simulink library "dragTurbine"  (R2022a)
settings: Solver=VariableStepAuto  StartTime=0.0  StopTime=10.0  RelTol=1e-3
undefined symbols (not defined in the file): flwSpd, rho, vcl
libraries: simulink x2, vrlib x2, localApparentWind_ul x1
settings Model: Creator=Ayaz  LastModifiedBy=kavin
settings SolverCC: AlgebraicLoopSolver=TrustRegion
settings DataIOCC: ReturnWorkspaceOutputs=off
settings DebuggingCC: UnconnectedInputMsg=warning  UnconnectedOutputMsg=warning  UnconnectedLineMsg=warning  SFMachineParentedDataDiag=warning  ArithmeticOperatorsInVariantConditions=warning
settings SFSimCC: CustomCodeUndefinedFunction=UseInterfaceOnly

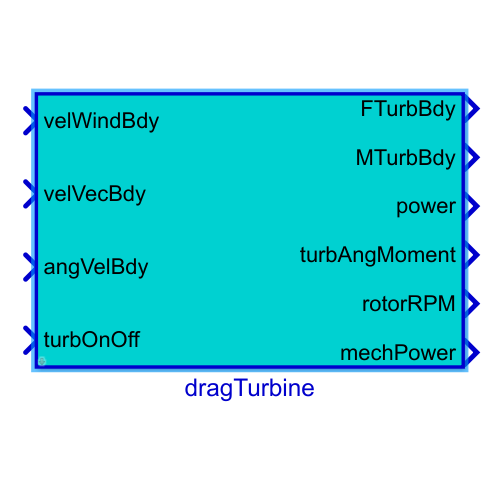
[thumbnail: Simulink's stored preview of the top-level diagram]
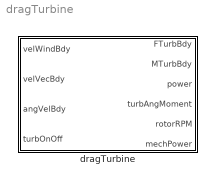
== system dragTurbine ==
  dragTurbine : Subsystem  TreatAsAtomicUnit=on  mask{vhcl=vcl, thr=0}
      mask prompts: vhcl "Vehicle Object"; thr "Tether Object"

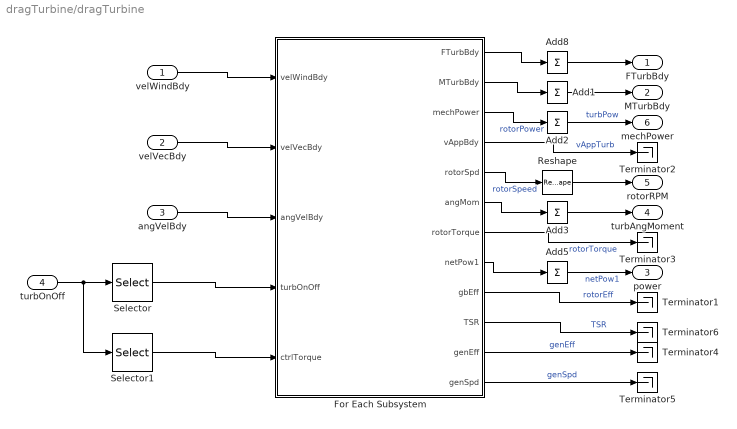
== system dragTurbine/dragTurbine ==
  velWindBdy : Inport
  velVecBdy : Inport  Port=2
  angVelBdy : Inport  Port=3
  turbOnOff : Inport  Port=4
  Add{1..3,8} (4 alike) : Sum  Inputs=1  CollapseMode=Specified dimension  CollapseDim=2
  Add5 : Sum  Inputs=1  CollapseDim=2
  For Each Subsystem : Subsystem  TreatAsAtomicUnit=on  mask{rho=rho, turb_struct=vhcl.struct('OCT.turb'), vhcl=vhcl}
      mask prompts: rho "Fluid Density"; turb_struct "Turbine Structure"; vhcl "Vehicle"
      settings: MinAlgLoopOccurrences=on
  Reshape : Reshape  OutputDimensionality=Column vector (2-D)
  Selector : Selector  InputPortWidth=1+vhcl.numTurbines.Value  IndexOptions=Index vector (dialog)  Indices=1  OutputSizes=1
  Selector1 : Selector  InputPortWidth=1+vhcl.numTurbines.Value  IndexOptions=Starting index (dialog)  Indices=2  OutputSizes=vhcl.numTurbines.Value
  Terminator{1..6} (6 alike) : Terminator
  FTurbBdy : Outport  PortDimensions=[3,1]  VectorParamsAs1DForOutWhenUnconnected=off
  MTurbBdy : Outport  Port=2  PortDimensions=[3,1]  VectorParamsAs1DForOutWhenUnconnected=off
  power : Outport  Port=3  PortDimensions=[1,1]  VectorParamsAs1DForOutWhenUnconnected=off
  turbAngMoment : Outport  Port=4  PortDimensions=[3,1]  VectorParamsAs1DForOutWhenUnconnected=off
  rotorRPM : Outport  Port=5  VectorParamsAs1DForOutWhenUnconnected=off
  mechPower : Outport  Port=6
  wires:
  velVecBdy/1 -> For Each Subsystem/2(velVecBdy)
  angVelBdy/1 -> For Each Subsystem/3(angVelBdy)
  turbOnOff/1 -> Selector1/1, Selector/1
  For Each Subsystem/1(FTurbBdy) -> Add8/1
  For Each Subsystem/2(MTurbBdy) -> Add1/1
  velWindBdy/1 -> For Each Subsystem/1(velWindBdy)
  Add8/1 -> FTurbBdy/1
  Add1/1 -> MTurbBdy/1
  For Each Subsystem/5(rotorSpd) -> Reshape/1  "rotorSpeed"
  For Each Subsystem/3(mechPower) -> Add2/1  "rotorPower"
  Add2/1 -> mechPower/1  "turbPow"
  For Each Subsystem/6(angMom) -> Add3/1
  Add3/1 -> turbAngMoment/1
  For Each Subsystem/4(vAppBdy) -> Terminator2/1  "vAppTurb"
  For Each Subsystem/7(rotorTorque) -> Terminator3/1  "rotorTorque"
  For Each Subsystem/9(gbEff) -> Terminator1/1  "rotorEff"
  For Each Subsystem/8(netPow1) -> Add5/1
  Add5/1 -> power/1  "netPow1"
  For Each Subsystem/10(TSR) -> Terminator6/1  "TSR"
  Selector1/1 -> For Each Subsystem/5(ctrlTorque)
  Selector/1 -> For Each Subsystem/4(turbOnOff)
  For Each Subsystem/11(genEff) -> Terminator4/1  "genEff"
  Reshape/1 -> rotorRPM/1
  For Each Subsystem/12(genSpd) -> Terminator5/1  "genSpd"

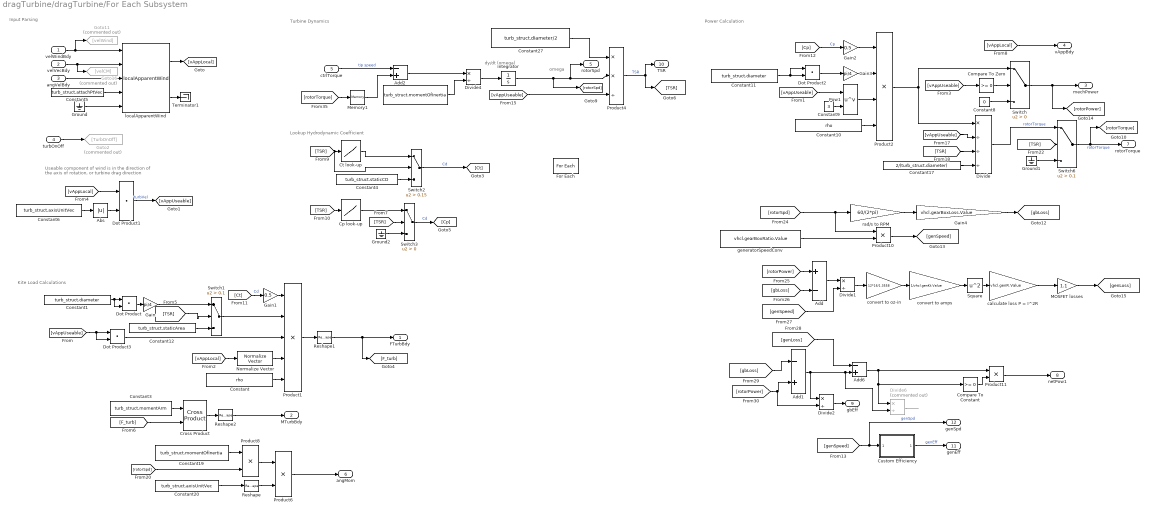
== system dragTurbine/dragTurbine/For Each Subsystem ==
  note: Lookup Hydrodynamic Coefficient
  note: Input Parsing
  note: Turbine Dynamics
  note: Kite Load Calculations
  note: Power Calculation
  note: Useable component of wind is in the direction of
      | the axis of rotation, or turbine drag direction
  note: dy/dt (omega)
  note: omega
  velWindBdy : Inport  Partition=on  PartitionDimension=2  PartitionWidth=1  PartitionOffset=0
  velVecBdy : Inport  Port=2
  angVelBdy : Inport  Port=3
  turbOnOff : Inport  Port=4
  ctrlTorque : Inport  Port=5  Partition=on  PartitionDimension=1  PartitionWidth=1  PartitionOffset=0
  " " : Constant  Value=turb_struct.momentOfInertia
  Abs : Abs  SaturateOnIntegerOverflow=off
  Add : Sum  Inputs=+-
  Add1 : Sum  Inputs=-+
  Add2 : Sum  Inputs=-+
  Add6 : Sum  Inputs=-+
  Compare To Constant : simulink/Logic and Bit Operations/Compare To Constant  relop=>=  const=0  OutDataTypeStr=boolean
  Compare To Zero : simulink/Logic and Bit Operations/Compare To Zero  relop=>=  OutDataTypeStr=boolean
  Constant : Constant  Value=rho
  Constant1 : Constant  Value=turb_struct.diameter  VectorParams1D=off
  Constant10 : Constant  Value=rho
  Constant11 : Constant  Value=turb_struct.diameter  VectorParams1D=off
  Constant12 : Constant  Value=turb_struct.staticArea  VectorParams1D=off
  Constant17 : Constant  Value=2/(turb_struct.diameter)
  Constant19 : Constant  Value=turb_struct.momentOfInertia
  Constant20 : Constant  Value=turb_struct.axisUnitVec
  Constant27 : Constant  Value=turb_struct.diameter/2
  Constant3 : Constant  Value=turb_struct.momentArm
  Constant4 : Constant  Value=turb_struct.staticCD
  Constant5 : Constant  Value=turb_struct.attachPtVec
  Constant6 : Constant  Value=turb_struct.axisUnitVec
  Constant8 : Constant  Value=0
  Constant9 : Constant  Value=3
  Cp look-up : Lookup_n-D  NumberOfTableDimensions=1  BreakpointsForDimension1=turb_struct.RPMref  Table=turb_struct.CpLookup  InternalRulePriority=Speed  RndMeth=Simplest
  Cross Product : vrlib/Utilities/Cross Product
  Ct look-up : Lookup_n-D  NumberOfTableDimensions=1  BreakpointsForDimension1=turb_struct.RPMref  Table=turb_struct.CtLookup  InternalRulePriority=Speed  RndMeth=Simplest
  Custom Efficiency : MATLAB Function  TreatAsAtomicUnit=on
  Divide : Product  Inputs=*///
  Divide1 : Product  Inputs=*/
  Divide2 : Product  Inputs=*/
  Divide4 : Product  Inputs=*/
  Divide6 : Product  Commented=on  Inputs=*/
  Dot Product{,1..3} (4 alike) : DotProduct  OutDataTypeStr=Inherit: Inherit via internal rule
  For Each : ForEach  DisableCoverage=on  IterateSubsysMaskParameter=off,on,off  SubsysMaskParameterIterationDimension=1,2,1  SubsysMaskParameterIterationStepSize=1,1,1
  Gain : Gain  Gain=pi/4
  Gain1 : Gain  Gain=0.5
  Gain2 : Gain  Gain=0.5
  Gain3 : Gain  Gain=pi/4
  Gain4 : Gain  Gain=vhcl.gearBoxLoss.Value
  Goto11 : Goto  Commented=on  GotoTag=velWind
  Goto16 : Goto  Commented=on  GotoTag=velCM
  Goto2 : Goto  Commented=on  GotoTag=TurbOnOff
  Ground : Ground
  Ground1 : Ground
  Ground2 : Ground
  Integrator : Integrator  InitialCondition=turb_struct.optTSR*(-vhcl.initVelVecBdy.Value(1)+flwSpd)/(turb_struct.diameter/2)
  MOSFET losses : Gain  Gain=1.1
  Memory1 : Memory  InitialCondition=10
  Normalize Vector : vrlib/Utilities/Normalize Vector  maxzero=0
  Pow1 : Math  Operator=pow  SignedPower=on  RndMeth=Zero
  Product1 : Product  Inputs=5
  Product{6,8,10..11} (4 alike) : Product
  Product2 : Product  Inputs=4
  Product4 : Product  Inputs=**/
  Reshape : Reshape  OutputDimensionality=Column vector (2-D)
  Reshape1 : Reshape  OutputDimensionality=Column vector (2-D)
  Reshape2 : Reshape  OutputDimensionality=Column vector (2-D)
  Square : Math  Operator=square
  Switch : Switch  Criteria=u2 > Threshold  SaturateOnIntegerOverflow=off  InputSameDT=off
  Switch1 : Switch  Criteria=u2 > Threshold  Threshold=0.1  SaturateOnIntegerOverflow=off  InputSameDT=off
  Switch2 : Switch  Criteria=u2 > Threshold  Threshold=0.15  SaturateOnIntegerOverflow=off  InputSameDT=off
  Switch3 : Switch  Criteria=u2 > Threshold  SaturateOnIntegerOverflow=off  InputSameDT=off
  Switch6 : Switch  Criteria=u2 > Threshold  Threshold=0.1  SaturateOnIntegerOverflow=off  InputSameDT=off
  Terminator1 : Terminator
  calculate loss P = I^2R : Gain  Gain=vhcl.genR.Value
  convert to amps : Gain  Gain=1/vhcl.genKt.Value
  convert to oz-in : Gain  Gain=12*16/1.3558
  generatorSpeedConv : Constant  Value=vhcl.gearBoxRatio.Value
  localApparentWind : localApparentWind_ul/localApparentWind  SystemSampleTime=-1  VariantActivationTime=update diagram  Latency=0  AutoFrameSizeCalculation=off
  rad/s to RPM : Gain  Gain=60/(2*pi)
  FTurbBdy : Outport  PortDimensions=[3,1]  ConcatenationDimension=2  VectorParamsAs1DForOutWhenUnconnected=off
  MTurbBdy : Outport  Port=2  PortDimensions=[3,1]  ConcatenationDimension=2  VectorParamsAs1DForOutWhenUnconnected=off
  mechPower : Outport  Port=3  PortDimensions=[1,1]  ConcatenationDimension=2  VectorParamsAs1DForOutWhenUnconnected=off
  vAppBdy : Outport  Port=4  PortDimensions=[3,1]  ConcatenationDimension=2  VectorParamsAs1DForOutWhenUnconnected=off
  rotorSpd : Outport  Port=5  ConcatenationDimension=2
  angMom : Outport  Port=6  ConcatenationDimension=2
  rotorTorque : Outport  Port=7  ConcatenationDimension=2
  netPow1 : Outport  Port=8  ConcatenationDimension=2
  gbEff : Outport  Port=9  ConcatenationDimension=2
  TSR : Outport  Port=10  ConcatenationDimension=2
  genEff : Outport  Port=11  ConcatenationDimension=2
  genSpd : Outport  Port=12  ConcatenationDimension=2
  wires:
  Gain2/1 -> Product2/1
  angVelBdy/1 -> localApparentWind/3
  Constant11/1 -> Dot Product2/2, Dot Product2/1
  [vAppUseable] -> Dot Product3/2, Dot Product3/1
  Constant10/1 -> Product2/4
  [vAppUseable] -> Pow1/1
  Dot Product2/1 -> Gain3/1
  [vAppLocal] -> Dot Product1/1
  Gain3/1 -> Product2/2
  Dot Product/1 -> Gain/1
  [vAppUseable] -> Compare To Zero/1
  Cross Product/1 -> Reshape2/1
  Constant8/1 -> Switch/3
  turbOnOff/1 -> Goto2/1
  Switch/1 -> [rotorPower], mechPower/1
  Gain1/1 -> Product1/1
  Gain/1 -> Switch1/1
  Pow1/1 -> Product2/3
  Constant9/1 -> Pow1/2
  Constant6/1 -> Abs/1
  Constant3/1 -> Cross Product/1
  Compare To Zero/1 -> Switch/2
  localApparentWind/1 -> [vAppLocal]
  Constant5/1 -> localApparentWind/4
  [vAppLocal] -> vAppBdy/1
  localApparentWind/2 -> Terminator1/1
  [Cp] -> Gain2/1  "Cp"
  Abs/1 -> Dot Product1/2
  [TSR] -> Divide/3
  [vAppLocal] -> Normalize Vector/1
  [TSR] -> Cp look-up/1
  Constant1/1 -> Dot Product/1, Dot Product/2
  velVecBdy/1 -> localApparentWind/2, Goto16/1
  Normalize Vector/1 -> Product1/4
  [TSR] -> Switch2/2, Ct look-up/1
  [Ct] -> Gain1/1  "Cd"
  [F_turb] -> Cross Product/2
  Switch2/1 -> [Ct]  "Cd"
  Constant12/1 -> Switch1/3
  Constant/1 -> Product1/5
  Dot Product3/1 -> Product1/3
  Product4/1 -> [TSR], TSR/1  "TSR"
  Constant4/1 -> Switch2/3
  Ct look-up/1 -> Switch2/1
  Ground/1 -> localApparentWind/5
  [vAppUseable] -> Divide/2
  Product1/1 -> Reshape1/1
  Switch1/1 -> Product1/2
  Switch6/1 -> [rotorTorque], rotorTorque/1  "rotorTorque"
  Product2/1 -> Switch/1, Divide/1
  Constant17/1 -> Divide/4
  Dot Product1/1 -> [vAppUseable]  "turbVel"
  [TSR] -> Switch1/2
  Constant20/1 -> Reshape/1
  Reshape/1 -> Product6/2
  Constant19/1 -> Product8/1
  Product8/1 -> Product6/1
  Gain4/1 -> [gbLoss]
  generatorSpeedConv/1 -> Product10/2
  Product10/1 -> [genSpeed]
  [gbLoss] -> Add/2
  [rotorPower] -> Add/1
  Add/1 -> Divide1/1
  [genSpeed] -> Divide1/2
  Divide1/1 -> convert to oz-in/1
  convert to oz-in/1 -> convert to amps/1
  convert to amps/1 -> Square/1
  Square/1 -> calculate loss P = I^2R/1
  calculate loss P = I^2R/1 -> MOSFET losses/1
  [gbLoss] -> Add1/1
  [genLoss] -> Add6/1
  [rotorPower] -> Add1/2, Divide2/2
  Product11/1 -> netPow1/1
  Compare To Constant/1 -> Product11/2
  Add6/1 -> Divide6/1, Compare To Constant/1, Product11/1
  Divide2/1 -> gbEff/1
  MOSFET losses/1 -> [genLoss]
  velWindBdy/1 -> localApparentWind/1, Goto11/1
  " "/1 -> Divide4/2
  Add2/1 -> Divide4/1
  Constant27/1 -> Product4/1
  Divide4/1 -> Integrator/1
  [rotorSpd] -> rad/s to RPM/1, Product10/1
  rad/s to RPM/1 -> Gain4/1
  Add1/1 -> Divide6/2, Add6/2, Divide2/1
  Divide6/1 -> ?
  [vAppUseable] -> Product4/3
  Cp look-up/1 -> Switch3/1
  [rotorSpd] -> Product8/2
  Product6/1 -> angMom/1
  Reshape1/1 -> FTurbBdy/1, [F_turb]
  Reshape2/1 -> MTurbBdy/1
  [rotorTorque] -> Memory1/1
  Divide/1 -> Switch6/1  "rotorTorque"
  [TSR] -> Switch6/2
  Ground1/1 -> Switch6/3
  ctrlTorque/1 -> Add2/1  "tip speed"
  Integrator/1 -> rotorSpd/1, Product4/2, [rotorSpd]
  Memory1/1 -> Add2/2
  [TSR] -> Switch3/2
  Ground2/1 -> Switch3/3
  Switch3/1 -> [Cp]  "Cd"
  [genSpeed] -> genSpd/1, Custom Efficiency/1(rotorSpeed)  "genSpd"
  Custom Efficiency/1(efficiency) -> genEff/1  "genEff"

== matlab function dragTurbine/For Each Subsystem/Custom Efficiency ==
  data: rotorSpeed input; efficiency output
function efficiency = generatorEfficiency(rotorSpeed)

efficiency = 0.5 + 0.2*(rotorSpeed^(0.15)) - 0.025*(rotorSpeed^(0.2));
